simulink library "inp"  (R2021b)
settings: Solver=VariableStepAuto  StartTime=0.0  StopTime=10.0  RelTol=1e-3
undefined symbols (not defined in the file): C_TASK_5MS_S, FALSE, KINP_AcoreReadyToSlp_flg_ovrdflg, KINP_AcoreReadyToSlp_flg_ovrdval, KINP_AllowMovThd_OTA_enum_ovrdflg, KINP_AllowMovThd_OTA_enum_ovrdval, KINP_APSAngleTarget_Deg_ovrdflg, KINP_APSAngleTarget_Deg_ovrdval, KINP_APSDecReq_mps2_ovrdflg, KINP_APSDecReq_mps2_ovrdval, KINP_APSDecReqA_flg_ovrdflg, KINP_APSDecReqA_flg_ovrdval, KINP_APSDFLL_cm_ovrdflg, KINP_APSDFLL_cm_ovrdval, KINP_APSDFLR_cm_ovrdflg, KINP_APSDFLR_cm_ovrdval, KINP_APSDRLL_cm_ovrdflg, KINP_APSDRLL_cm_ovrdval, KINP_APSDRLR_cm_ovrdflg, KINP_APSDRLR_cm_ovrdval, KINP_APSExitCondition_enum_ovrdflg, KINP_APSExitCondition_enum_ovrdval, KINP_APSHWVer_enum_ovrdflg, KINP_APSHWVer_enum_ovrdval, KINP_APSProgressPCT_pct_ovrdflg, KINP_APSProgressPCT_pct_ovrdval, KINP_APSReq_enum_ovrdflg, KINP_APSReq_enum_ovrdval, KINP_APSRQDisplay_enum_ovrdflg, KINP_APSRQDisplay_enum_ovrdval, KINP_APSRqEPASCtrl_flg_ovrdflg, KINP_APSRqEPASCtrl_flg_ovrdval, KINP_APSShiftPosnReq_enum_ovrdval, KINP_APSShiftPosnReq_enum_ovrflg, KINP_APSSpeedCMD_kph_ovrdval, KINP_APSSpeedCMD_kph_ovrflg, KINP_APSStaSystem_enum_ovrdflg, KINP_APSStaSystem_enum_ovrdval, KINP_APSSWVer_enum_ovrdflg, KINP_APSSWVer_enum_ovrdval, KINP_APSVMCReqA_flg_ovrdval, KINP_APSVMCReqA_flg_ovrflg, KINP_APSVRqEPASCtrl_flg_ovrdflg, KINP_APSVRqEPASCtrl_flg_ovrdval, KINP_AuxBattVolmV_mV_ovrdflg, KINP_AuxBattVolmV_mV_ovrdval, KINP_CAASSta_enum_ovrdflg, KINP_CAASSta_enum_ovrdval, KINP_CAASVMCReqA_flg_ovrdval, KINP_CAASVMCReqA_flg_ovrflg, KINP_Chime_enum_ovrdflg, KINP_Chime_enum_ovrdval, KINP_ClearDTCcmd_flg_ovrdflg, KINP_ClearDTCcmd_flg_ovrdval, KINP_EvccAplusPwrUpReq_flg_ovrdflg, KINP_EvccAplusPwrUpReq_flg_ovrdval, KINP_LFID_raw_ovrdval, KINP_LFID_raw_ovrflg, KINP_LRID_raw_ovrdval, KINP_MemOffsetAccX_raw16_ovrdflg ... (+118)
libraries: FVT_lib x942, hcu_lib x1
(part 16 of 31)

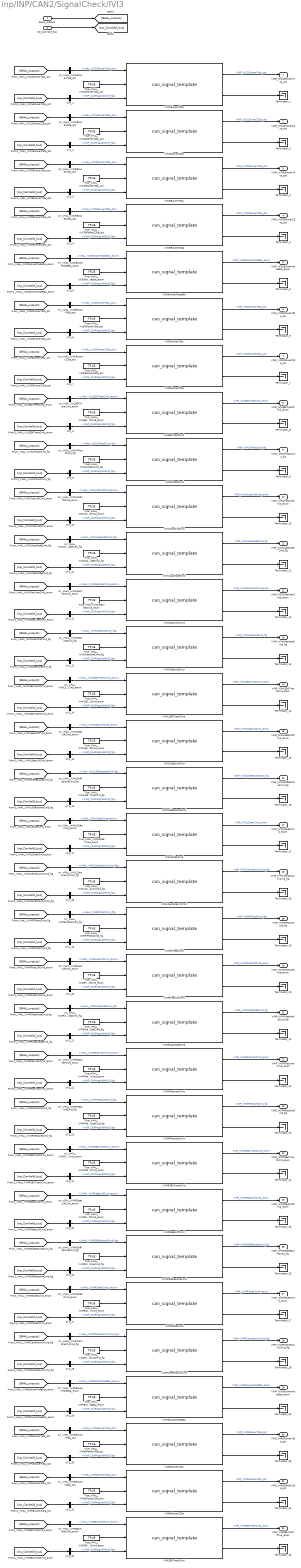
== system inp/INP/CAN2/SignalCheck/IVI3 ==
  BHAL_outputs : Inport
  inp_CanValid_bus : Inport  Port=2
  IVICLBlowerYSta : FVT_lib/inp/can_signal_template  SystemSampleTime=-1  VariantActivationTime=update diagram  Latency=0  AutoFrameSizeCalculation=off
      link override defval: Value=KINP_IVICLBlowerYSta_pct_defval
      link override ovrdflg: Value=KINP_IVICLBlowerYSta_pct_ovrdflg
      link override ovrdval: Value=KINP_IVICLBlowerYSta_pct_ovrdval
  IVICLBlowerZSta : FVT_lib/inp/can_signal_template  SystemSampleTime=-1  VariantActivationTime=update diagram  Latency=0  AutoFrameSizeCalculation=off
      link override defval: Value=KINP_IVICLBlowerZSta_pct_defval
      link override ovrdflg: Value=KINP_IVICLBlowerZSta_pct_ovrdflg
      link override ovrdval: Value=KINP_IVICLBlowerZSta_pct_ovrdval
  IVICRBlowerYSta : FVT_lib/inp/can_signal_template  SystemSampleTime=-1  VariantActivationTime=update diagram  Latency=0  AutoFrameSizeCalculation=off
      link override defval: Value=KINP_IVICRBlowerYSta_pct_defval
      link override ovrdflg: Value=KINP_IVICRBlowerYSta_pct_ovrdflg
      link override ovrdval: Value=KINP_IVICRBlowerYSta_pct_ovrdval
  IVICRBlowerZSta : FVT_lib/inp/can_signal_template  SystemSampleTime=-1  VariantActivationTime=update diagram  Latency=0  AutoFrameSizeCalculation=off
      link override defval: Value=KINP_IVICRBlowerZSta_pct_defval
      link override ovrdflg: Value=KINP_IVICRBlowerZSta_pct_ovrdflg
      link override ovrdval: Value=KINP_IVICRBlowerZSta_pct_ovrdval
  IVIDrBlowerModeSta : FVT_lib/inp/can_signal_template  SystemSampleTime=-1  VariantActivationTime=update diagram  Latency=0  AutoFrameSizeCalculation=off
      link override defval: Value=KINP_IVIDrBlowerModeSta_enum_defval
      link override ovrdflg: Value=KINP_IVIDrBlowerModeSta_enum_ovrdflg
      link override ovrdval: Value=KINP_IVIDrBlowerModeSta_enum_ovrdval
  IVIDrBlowerYSta : FVT_lib/inp/can_signal_template  SystemSampleTime=-1  VariantActivationTime=update diagram  Latency=0  AutoFrameSizeCalculation=off
      link override defval: Value=KINP_IVIDrBlowerYSta_pct_defval
      link override ovrdflg: Value=KINP_IVIDrBlowerYSta_pct_ovrdflg
      link override ovrdval: Value=KINP_IVIDrBlowerYSta_pct_ovrdval
  IVIDrBlowerZSta : FVT_lib/inp/can_signal_template  SystemSampleTime=-1  VariantActivationTime=update diagram  Latency=0  AutoFrameSizeCalculation=off
      link override defval: Value=KINP_IVIDrBlowerZSta_pct_defval
      link override ovrdflg: Value=KINP_IVIDrBlowerZSta_pct_ovrdflg
      link override ovrdval: Value=KINP_IVIDrBlowerZSta_pct_ovrdval
  IVILSEATventCmd : FVT_lib/inp/can_signal_template  SystemSampleTime=-1  VariantActivationTime=update diagram  Latency=0  AutoFrameSizeCalculation=off
      link override defval: Value=KINP_IVILSEATventCmd_enum_defval
      link override ovrdflg: Value=KINP_IVILSEATventCmd_enum_ovrdflg
      link override ovrdval: Value=KINP_IVILSEATventCmd_enum_ovrdval
  IVIMLFMostCmd : FVT_lib/inp/can_signal_template  SystemSampleTime=-1  VariantActivationTime=update diagram  Latency=0  AutoFrameSizeCalculation=off
      link override defval: Value=KINP_IVIMLFMostCmd_flg_defval
      link override ovrdflg: Value=KINP_IVIMLFMostCmd_flg_ovrdflg
      link override ovrdval: Value=KINP_IVIMLFMostCmd_flg_ovrdval
  IVIMLFootLiftCmd : FVT_lib/inp/can_signal_template  SystemSampleTime=-1  VariantActivationTime=update diagram  Latency=0  AutoFrameSizeCalculation=off
      link override defval: Value=KINP_IVIMLFootLiftCmd_enum_defval
      link override ovrdflg: Value=KINP_IVIMLFootLiftCmd_enum_ovrdflg
      link override ovrdval: Value=KINP_IVIMLFootLiftCmd_enum_ovrdval
  IVIMLNapModeCmd : FVT_lib/inp/can_signal_template  SystemSampleTime=-1  VariantActivationTime=update diagram  Latency=0  AutoFrameSizeCalculation=off
      link override defval: Value=KINP_IVIMLNapModeCmd_flg_defval
      link override ovrdflg: Value=KINP_IVIMLNapModeCmd_flg_ovrdflg
      link override ovrdval: Value=KINP_IVIMLNapModeCmd_flg_ovrdval
  IVIMLReclinerCmd : FVT_lib/inp/can_signal_template  SystemSampleTime=-1  VariantActivationTime=update diagram  Latency=0  AutoFrameSizeCalculation=off
      link override defval: Value=KINP_IVIMLReclinerCmd_enum_defval
      link override ovrdflg: Value=KINP_IVIMLReclinerCmd_enum_ovrdflg
      link override ovrdval: Value=KINP_IVIMLReclinerCmd_enum_ovrdval
  IVIMLRestoreCmd : FVT_lib/inp/can_signal_template  SystemSampleTime=-1  VariantActivationTime=update diagram  Latency=0  AutoFrameSizeCalculation=off
      link override defval: Value=KINP_IVIMLRestoreCmd_flg_defval
      link override ovrdflg: Value=KINP_IVIMLRestoreCmd_flg_ovrdflg
      link override ovrdval: Value=KINP_IVIMLRestoreCmd_flg_ovrdval
  IVIMLSEATventCmd : FVT_lib/inp/can_signal_template  SystemSampleTime=-1  VariantActivationTime=update diagram  Latency=0  AutoFrameSizeCalculation=off
      link override defval: Value=KINP_IVIMLSEATventCmd_enum_defval
      link override ovrdflg: Value=KINP_IVIMLSEATventCmd_enum_ovrdflg
      link override ovrdval: Value=KINP_IVIMLSEATventCmd_enum_ovrdval
  IVIMLSeatLiftCmd : FVT_lib/inp/can_signal_template  SystemSampleTime=-1  VariantActivationTime=update diagram  Latency=0  AutoFrameSizeCalculation=off
      link override defval: Value=KINP_IVIMLSeatLiftCmd_enum_defval
      link override ovrdflg: Value=KINP_IVIMLSeatLiftCmd_enum_ovrdflg
      link override ovrdval: Value=KINP_IVIMLSeatLiftCmd_enum_ovrdval
  IVIMLSldRestoreCmd : FVT_lib/inp/can_signal_template  SystemSampleTime=-1  VariantActivationTime=update diagram  Latency=0  AutoFrameSizeCalculation=off
      link override defval: Value=KINP_IVIMLSldRestoreCmd_flg_defval
      link override ovrdflg: Value=KINP_IVIMLSldRestoreCmd_flg_ovrdflg
      link override ovrdval: Value=KINP_IVIMLSldRestoreCmd_flg_ovrdval
  IVIMLSliderCmd : FVT_lib/inp/can_signal_template  SystemSampleTime=-1  VariantActivationTime=update diagram  Latency=0  AutoFrameSizeCalculation=off
      link override defval: Value=KINP_IVIMLSliderCmd_enum_defval
      link override ovrdflg: Value=KINP_IVIMLSliderCmd_enum_ovrdflg
      link override ovrdval: Value=KINP_IVIMLSliderCmd_enum_ovrdval
  IVIMLZeroGravityCmd : FVT_lib/inp/can_signal_template  SystemSampleTime=-1  VariantActivationTime=update diagram  Latency=0  AutoFrameSizeCalculation=off
      link override defval: Value=KINP_IVIMLZeroGravityCmd_flg_defval
      link override ovrdflg: Value=KINP_IVIMLZeroGravityCmd_flg_ovrdflg
      link override ovrdval: Value=KINP_IVIMLZeroGravityCmd_flg_ovrdval
  IVIMRFMostCmd : FVT_lib/inp/can_signal_template  SystemSampleTime=-1  VariantActivationTime=update diagram  Latency=0  AutoFrameSizeCalculation=off
      link override defval: Value=KINP_IVIMRFMostCmd_flg_defval
      link override ovrdflg: Value=KINP_IVIMRFMostCmd_flg_ovrdflg
      link override ovrdval: Value=KINP_IVIMRFMostCmd_flg_ovrdval
  IVIMRFootLiftCmd : FVT_lib/inp/can_signal_template  SystemSampleTime=-1  VariantActivationTime=update diagram  Latency=0  AutoFrameSizeCalculation=off
      link override defval: Value=KINP_IVIMRFootLiftCmd_enum_defval
      link override ovrdflg: Value=KINP_IVIMRFootLiftCmd_enum_ovrdflg
      link override ovrdval: Value=KINP_IVIMRFootLiftCmd_enum_ovrdval
  IVIMRNapModeCmd : FVT_lib/inp/can_signal_template  SystemSampleTime=-1  VariantActivationTime=update diagram  Latency=0  AutoFrameSizeCalculation=off
      link override defval: Value=KINP_IVIMRNapModeCmd_flg_defval
      link override ovrdflg: Value=KINP_IVIMRNapModeCmd_flg_ovrdflg
      link override ovrdval: Value=KINP_IVIMRNapModeCmd_flg_ovrdval
  IVIMRReclinerCmd : FVT_lib/inp/can_signal_template  SystemSampleTime=-1  VariantActivationTime=update diagram  Latency=0  AutoFrameSizeCalculation=off
      link override defval: Value=KINP_IVIMRReclinerCmd_enum_defval
      link override ovrdflg: Value=KINP_IVIMRReclinerCmd_enum_ovrdflg
      link override ovrdval: Value=KINP_IVIMRReclinerCmd_enum_ovrdval
  IVIMRRestoreCmd : FVT_lib/inp/can_signal_template  SystemSampleTime=-1  VariantActivationTime=update diagram  Latency=0  AutoFrameSizeCalculation=off
      link override defval: Value=KINP_IVIMRRestoreCmd_flg_defval
      link override ovrdflg: Value=KINP_IVIMRRestoreCmd_flg_ovrdflg
      link override ovrdval: Value=KINP_IVIMRRestoreCmd_flg_ovrdval
  IVIMRSEATventCmd : FVT_lib/inp/can_signal_template  SystemSampleTime=-1  VariantActivationTime=update diagram  Latency=0  AutoFrameSizeCalculation=off
      link override defval: Value=KINP_IVIMRSEATventCmd_enum_defval
      link override ovrdflg: Value=KINP_IVIMRSEATventCmd_enum_ovrdflg
      link override ovrdval: Value=KINP_IVIMRSEATventCmd_enum_ovrdval
  IVIMRSeatLiftCmd : FVT_lib/inp/can_signal_template  SystemSampleTime=-1  VariantActivationTime=update diagram  Latency=0  AutoFrameSizeCalculation=off
      link override defval: Value=KINP_IVIMRSeatLiftCmd_enum_defval
      link override ovrdflg: Value=KINP_IVIMRSeatLiftCmd_enum_ovrdflg
      link override ovrdval: Value=KINP_IVIMRSeatLiftCmd_enum_ovrdval
  IVIMRSldRestoreCmd : FVT_lib/inp/can_signal_template  SystemSampleTime=-1  VariantActivationTime=update diagram  Latency=0  AutoFrameSizeCalculation=off
      link override defval: Value=KINP_IVIMRSldRestoreCmd_flg_defval
      link override ovrdflg: Value=KINP_IVIMRSldRestoreCmd_flg_ovrdflg
      link override ovrdval: Value=KINP_IVIMRSldRestoreCmd_flg_ovrdval
  IVIMRSliderCmd : FVT_lib/inp/can_signal_template  SystemSampleTime=-1  VariantActivationTime=update diagram  Latency=0  AutoFrameSizeCalculation=off
      link override defval: Value=KINP_IVIMRSliderCmd_enum_defval
      link override ovrdflg: Value=KINP_IVIMRSliderCmd_enum_ovrdflg
      link override ovrdval: Value=KINP_IVIMRSliderCmd_enum_ovrdval
  IVIMRZeroGravityCmd : FVT_lib/inp/can_signal_template  SystemSampleTime=-1  VariantActivationTime=update diagram  Latency=0  AutoFrameSizeCalculation=off
      link override defval: Value=KINP_IVIMRZeroGravityCmd_flg_defval
      link override ovrdflg: Value=KINP_IVIMRZeroGravityCmd_flg_ovrdflg
      link override ovrdval: Value=KINP_IVIMRZeroGravityCmd_flg_ovrdval
  IVIPsBlowerModeSta : FVT_lib/inp/can_signal_template  SystemSampleTime=-1  VariantActivationTime=update diagram  Latency=0  AutoFrameSizeCalculation=off
      link override defval: Value=KINP_IVIPsBlowerModeSta_enum_defval
      link override ovrdflg: Value=KINP_IVIPsBlowerModeSta_enum_ovrdflg
      link override ovrdval: Value=KINP_IVIPsBlowerModeSta_enum_ovrdval
  IVIPsBlowerYSta : FVT_lib/inp/can_signal_template  SystemSampleTime=-1  VariantActivationTime=update diagram  Latency=0  AutoFrameSizeCalculation=off
      link override defval: Value=KINP_IVIPsBlowerYSta_pct_defval
      link override ovrdflg: Value=KINP_IVIPsBlowerYSta_pct_ovrdflg
      link override ovrdval: Value=KINP_IVIPsBlowerYSta_pct_ovrdval
  IVIPsBlowerZSta : FVT_lib/inp/can_signal_template  SystemSampleTime=-1  VariantActivationTime=update diagram  Latency=0  AutoFrameSizeCalculation=off
      link override defval: Value=KINP_IVIPsBlowerZSta_pct_defval
      link override ovrdflg: Value=KINP_IVIPsBlowerZSta_pct_ovrdflg
      link override ovrdval: Value=KINP_IVIPsBlowerZSta_pct_ovrdval
  IVIRSEATventCmd : FVT_lib/inp/can_signal_template  SystemSampleTime=-1  VariantActivationTime=update diagram  Latency=0  AutoFrameSizeCalculation=off
      link override defval: Value=KINP_IVIRSEATventCmd_enum_defval
      link override ovrdflg: Value=KINP_IVIRSEATventCmd_enum_ovrdflg
      link override ovrdval: Value=KINP_IVIRSEATventCmd_enum_ovrdval
  Terminator_{1..32} (32 alike) : Terminator
  True_VHAL_IVICLBlowerYSta_pct : Constant  Value=TRUE  OutDataTypeStr=boolean
  True_VHAL_IVICLBlowerZSta_pct : Constant  Value=TRUE  OutDataTypeStr=boolean
  True_VHAL_IVICRBlowerYSta_pct : Constant  Value=TRUE  OutDataTypeStr=boolean
  True_VHAL_IVICRBlowerZSta_pct : Constant  Value=TRUE  OutDataTypeStr=boolean
  True_VHAL_IVIDrBlowerModeSta_enum : Constant  Value=TRUE  OutDataTypeStr=boolean
  True_VHAL_IVIDrBlowerYSta_pct : Constant  Value=TRUE  OutDataTypeStr=boolean
  True_VHAL_IVIDrBlowerZSta_pct : Constant  Value=TRUE  OutDataTypeStr=boolean
  True_VHAL_IVILSEATventCmd_enum : Constant  Value=TRUE  OutDataTypeStr=boolean
  True_VHAL_IVIMLFMostCmd_flg : Constant  Value=TRUE  OutDataTypeStr=boolean
  True_VHAL_IVIMLFootLiftCmd_enum : Constant  Value=TRUE  OutDataTypeStr=boolean
  True_VHAL_IVIMLNapModeCmd_flg : Constant  Value=TRUE  OutDataTypeStr=boolean
  True_VHAL_IVIMLReclinerCmd_enum : Constant  Value=TRUE  OutDataTypeStr=boolean
  True_VHAL_IVIMLRestoreCmd_flg : Constant  Value=TRUE  OutDataTypeStr=boolean
  True_VHAL_IVIMLSEATventCmd_enum : Constant  Value=TRUE  OutDataTypeStr=boolean
  True_VHAL_IVIMLSeatLiftCmd_enum : Constant  Value=TRUE  OutDataTypeStr=boolean
  True_VHAL_IVIMLSldRestoreCmd_flg : Constant  Value=TRUE  OutDataTypeStr=boolean
  True_VHAL_IVIMLSliderCmd_enum : Constant  Value=TRUE  OutDataTypeStr=boolean
  True_VHAL_IVIMLZeroGravityCmd_flg : Constant  Value=TRUE  OutDataTypeStr=boolean
  True_VHAL_IVIMRFMostCmd_flg : Constant  Value=TRUE  OutDataTypeStr=boolean
  True_VHAL_IVIMRFootLiftCmd_enum : Constant  Value=TRUE  OutDataTypeStr=boolean
  True_VHAL_IVIMRNapModeCmd_flg : Constant  Value=TRUE  OutDataTypeStr=boolean
  True_VHAL_IVIMRReclinerCmd_enum : Constant  Value=TRUE  OutDataTypeStr=boolean
  True_VHAL_IVIMRRestoreCmd_flg : Constant  Value=TRUE  OutDataTypeStr=boolean
  True_VHAL_IVIMRSEATventCmd_enum : Constant  Value=TRUE  OutDataTypeStr=boolean
  True_VHAL_IVIMRSeatLiftCmd_enum : Constant  Value=TRUE  OutDataTypeStr=boolean
  True_VHAL_IVIMRSldRestoreCmd_flg : Constant  Value=TRUE  OutDataTypeStr=boolean
  True_VHAL_IVIMRSliderCmd_enum : Constant  Value=TRUE  OutDataTypeStr=boolean
  True_VHAL_IVIMRZeroGravityCmd_flg : Constant  Value=TRUE  OutDataTypeStr=boolean
  True_VHAL_IVIPsBlowerModeSta_enum : Constant  Value=TRUE  OutDataTypeStr=boolean
  True_VHAL_IVIPsBlowerYSta_pct : Constant  Value=TRUE  OutDataTypeStr=boolean
  True_VHAL_IVIPsBlowerZSta_pct : Constant  Value=TRUE  OutDataTypeStr=boolean
  True_VHAL_IVIRSEATventCmd_enum : Constant  Value=TRUE  OutDataTypeStr=boolean
  slr1_{1..32} (32 alike) : BusSelector  OutputSignals=VINP_CANMsgValidIVI3_flg
  slr_VHAL_IVICLBlowerYSta_pct : BusSelector  OutputSignals=VHAL_IVICLBlowerYSta_pct
  slr_VHAL_IVICLBlowerZSta_pct : BusSelector  OutputSignals=VHAL_IVICLBlowerZSta_pct
  slr_VHAL_IVICRBlowerYSta_pct : BusSelector  OutputSignals=VHAL_IVICRBlowerYSta_pct
  slr_VHAL_IVICRBlowerZSta_pct : BusSelector  OutputSignals=VHAL_IVICRBlowerZSta_pct
  slr_VHAL_IVIDrBlowerModeSta_enum : BusSelector  OutputSignals=VHAL_IVIDrBlowerModeSta_enum
  slr_VHAL_IVIDrBlowerYSta_pct : BusSelector  OutputSignals=VHAL_IVIDrBlowerYSta_pct
  slr_VHAL_IVIDrBlowerZSta_pct : BusSelector  OutputSignals=VHAL_IVIDrBlowerZSta_pct
  slr_VHAL_IVILSEATventCmd_enum : BusSelector  OutputSignals=VHAL_IVILSEATventCmd_enum
  slr_VHAL_IVIMLFMostCmd_flg : BusSelector  OutputSignals=VHAL_IVIMLFMostCmd_flg
  slr_VHAL_IVIMLFootLiftCmd_enum : BusSelector  OutputSignals=VHAL_IVIMLFootLiftCmd_enum
  slr_VHAL_IVIMLNapModeCmd_flg : BusSelector  OutputSignals=VHAL_IVIMLNapModeCmd_flg
  slr_VHAL_IVIMLReclinerCmd_enum : BusSelector  OutputSignals=VHAL_IVIMLReclinerCmd_enum
  slr_VHAL_IVIMLRestoreCmd_flg : BusSelector  OutputSignals=VHAL_IVIMLRestoreCmd_flg
  slr_VHAL_IVIMLSEATventCmd_enum : BusSelector  OutputSignals=VHAL_IVIMLSEATventCmd_enum
  slr_VHAL_IVIMLSeatLiftCmd_enum : BusSelector  OutputSignals=VHAL_IVIMLSeatLiftCmd_enum
  slr_VHAL_IVIMLSldRestoreCmd_flg : BusSelector  OutputSignals=VHAL_IVIMLSldRestoreCmd_flg
  slr_VHAL_IVIMLSliderCmd_enum : BusSelector  OutputSignals=VHAL_IVIMLSliderCmd_enum
  slr_VHAL_IVIMLZeroGravityCmd_flg : BusSelector  OutputSignals=VHAL_IVIMLZeroGravityCmd_flg
  slr_VHAL_IVIMRFMostCmd_flg : BusSelector  OutputSignals=VHAL_IVIMRFMostCmd_flg
  slr_VHAL_IVIMRFootLiftCmd_enum : BusSelector  OutputSignals=VHAL_IVIMRFootLiftCmd_enum
  slr_VHAL_IVIMRNapModeCmd_flg : BusSelector  OutputSignals=VHAL_IVIMRNapModeCmd_flg
  slr_VHAL_IVIMRReclinerCmd_enum : BusSelector  OutputSignals=VHAL_IVIMRReclinerCmd_enum
  slr_VHAL_IVIMRRestoreCmd_flg : BusSelector  OutputSignals=VHAL_IVIMRRestoreCmd_flg
  slr_VHAL_IVIMRSEATventCmd_enum : BusSelector  OutputSignals=VHAL_IVIMRSEATventCmd_enum
  slr_VHAL_IVIMRSeatLiftCmd_enum : BusSelector  OutputSignals=VHAL_IVIMRSeatLiftCmd_enum
  slr_VHAL_IVIMRSldRestoreCmd_flg : BusSelector  OutputSignals=VHAL_IVIMRSldRestoreCmd_flg
  slr_VHAL_IVIMRSliderCmd_enum : BusSelector  OutputSignals=VHAL_IVIMRSliderCmd_enum
  slr_VHAL_IVIMRZeroGravityCmd_flg : BusSelector  OutputSignals=VHAL_IVIMRZeroGravityCmd_flg
  slr_VHAL_IVIPsBlowerModeSta_enum : BusSelector  OutputSignals=VHAL_IVIPsBlowerModeSta_enum
  slr_VHAL_IVIPsBlowerYSta_pct : BusSelector  OutputSignals=VHAL_IVIPsBlowerYSta_pct
  slr_VHAL_IVIPsBlowerZSta_pct : BusSelector  OutputSignals=VHAL_IVIPsBlowerZSta_pct
  slr_VHAL_IVIRSEATventCmd_enum : BusSelector  OutputSignals=VHAL_IVIRSEATventCmd_enum
  VINP_IVICLBlowerYSta_pct : Outport
  VINP_IVICLBlowerZSta_pct : Outport  Port=2
  VINP_IVICRBlowerYSta_pct : Outport  Port=3
  VINP_IVICRBlowerZSta_pct : Outport  Port=4
  VINP_IVIDrBlowerModeSta_enum : Outport  Port=5
  VINP_IVIDrBlowerYSta_pct : Outport  Port=6
  VINP_IVIDrBlowerZSta_pct : Outport  Port=7
  VINP_IVILSEATventCmd_enum : Outport  Port=8
  VINP_IVIMLFMostCmd_flg : Outport  Port=9
  VINP_IVIMLFootLiftCmd_enum : Outport  Port=10
  VINP_IVIMLNapModeCmd_flg : Outport  Port=11
  VINP_IVIMLReclinerCmd_enum : Outport  Port=12
  VINP_IVIMLRestoreCmd_flg : Outport  Port=13
  VINP_IVIMLSEATventCmd_enum : Outport  Port=14
  VINP_IVIMLSeatLiftCmd_enum : Outport  Port=15
  VINP_IVIMLSldRestoreCmd_flg : Outport  Port=16
  VINP_IVIMLSliderCmd_enum : Outport  Port=17
  VINP_IVIMLZeroGravityCmd_flg : Outport  Port=18
  VINP_IVIMRFMostCmd_flg : Outport  Port=19
  VINP_IVIMRFootLiftCmd_enum : Outport  Port=20
  VINP_IVIMRNapModeCmd_flg : Outport  Port=21
  VINP_IVIMRReclinerCmd_enum : Outport  Port=22
  VINP_IVIMRRestoreCmd_flg : Outport  Port=23
  VINP_IVIMRSEATventCmd_enum : Outport  Port=24
  VINP_IVIMRSeatLiftCmd_enum : Outport  Port=25
  VINP_IVIMRSldRestoreCmd_flg : Outport  Port=26
  VINP_IVIMRSliderCmd_enum : Outport  Port=27
  VINP_IVIMRZeroGravityCmd_flg : Outport  Port=28
  VINP_IVIPsBlowerModeSta_enum : Outport  Port=29
  VINP_IVIPsBlowerYSta_pct : Outport  Port=30
  VINP_IVIPsBlowerZSta_pct : Outport  Port=31
  VINP_IVIRSEATventCmd_enum : Outport  Port=32
  wires:
  BHAL_outputs/1 -> [BHAL_outputs]
  inp_CanValid_bus/1 -> [inp_CanValid_bus]
  [BHAL_outputs] -> slr_VHAL_IVICLBlowerYSta_pct/1
  slr_VHAL_IVICLBlowerYSta_pct/1 -> IVICLBlowerYSta/1  "<VHAL_IVICLBlowerYSta_pct>"
  True_VHAL_IVICLBlowerYSta_pct/1 -> IVICLBlowerYSta/2
  [inp_CanValid_bus] -> slr1_1/1
  slr1_1/1 -> IVICLBlowerYSta/3  "<VINP_CANMsgValidIVI3_flg>"
  IVICLBlowerYSta/1 -> VINP_IVICLBlowerYSta_pct/1  "VINP_IVICLBlowerYSta_pct"
  IVICLBlowerYSta/2 -> Terminator_1/1
  [BHAL_outputs] -> slr_VHAL_IVICLBlowerZSta_pct/1
  slr_VHAL_IVICLBlowerZSta_pct/1 -> IVICLBlowerZSta/1  "<VHAL_IVICLBlowerZSta_pct>"
  True_VHAL_IVICLBlowerZSta_pct/1 -> IVICLBlowerZSta/2
  [inp_CanValid_bus] -> slr1_2/1
  slr1_2/1 -> IVICLBlowerZSta/3  "<VINP_CANMsgValidIVI3_flg>"
  IVICLBlowerZSta/1 -> VINP_IVICLBlowerZSta_pct/1  "VINP_IVICLBlowerZSta_pct"
  IVICLBlowerZSta/2 -> Terminator_2/1
  [BHAL_outputs] -> slr_VHAL_IVICRBlowerYSta_pct/1
  slr_VHAL_IVICRBlowerYSta_pct/1 -> IVICRBlowerYSta/1  "<VHAL_IVICRBlowerYSta_pct>"
  True_VHAL_IVICRBlowerYSta_pct/1 -> IVICRBlowerYSta/2
  [inp_CanValid_bus] -> slr1_3/1
  slr1_3/1 -> IVICRBlowerYSta/3  "<VINP_CANMsgValidIVI3_flg>"
  IVICRBlowerYSta/1 -> VINP_IVICRBlowerYSta_pct/1  "VINP_IVICRBlowerYSta_pct"
  IVICRBlowerYSta/2 -> Terminator_3/1
  [BHAL_outputs] -> slr_VHAL_IVICRBlowerZSta_pct/1
  slr_VHAL_IVICRBlowerZSta_pct/1 -> IVICRBlowerZSta/1  "<VHAL_IVICRBlowerZSta_pct>"
  True_VHAL_IVICRBlowerZSta_pct/1 -> IVICRBlowerZSta/2
  [inp_CanValid_bus] -> slr1_4/1
  slr1_4/1 -> IVICRBlowerZSta/3  "<VINP_CANMsgValidIVI3_flg>"
  IVICRBlowerZSta/1 -> VINP_IVICRBlowerZSta_pct/1  "VINP_IVICRBlowerZSta_pct"
  IVICRBlowerZSta/2 -> Terminator_4/1
  [BHAL_outputs] -> slr_VHAL_IVIDrBlowerModeSta_enum/1
  slr_VHAL_IVIDrBlowerModeSta_enum/1 -> IVIDrBlowerModeSta/1  "<VHAL_IVIDrBlowerModeSta_enum>"
  True_VHAL_IVIDrBlowerModeSta_enum/1 -> IVIDrBlowerModeSta/2
  [inp_CanValid_bus] -> slr1_5/1
  slr1_5/1 -> IVIDrBlowerModeSta/3  "<VINP_CANMsgValidIVI3_flg>"
  IVIDrBlowerModeSta/1 -> VINP_IVIDrBlowerModeSta_enum/1  "VINP_IVIDrBlowerModeSta_enum"
  IVIDrBlowerModeSta/2 -> Terminator_5/1
  [BHAL_outputs] -> slr_VHAL_IVIDrBlowerYSta_pct/1
  slr_VHAL_IVIDrBlowerYSta_pct/1 -> IVIDrBlowerYSta/1  "<VHAL_IVIDrBlowerYSta_pct>"
  True_VHAL_IVIDrBlowerYSta_pct/1 -> IVIDrBlowerYSta/2
  [inp_CanValid_bus] -> slr1_6/1
  slr1_6/1 -> IVIDrBlowerYSta/3  "<VINP_CANMsgValidIVI3_flg>"
  IVIDrBlowerYSta/1 -> VINP_IVIDrBlowerYSta_pct/1  "VINP_IVIDrBlowerYSta_pct"
  IVIDrBlowerYSta/2 -> Terminator_6/1
  [BHAL_outputs] -> slr_VHAL_IVIDrBlowerZSta_pct/1
  slr_VHAL_IVIDrBlowerZSta_pct/1 -> IVIDrBlowerZSta/1  "<VHAL_IVIDrBlowerZSta_pct>"
  True_VHAL_IVIDrBlowerZSta_pct/1 -> IVIDrBlowerZSta/2
  [inp_CanValid_bus] -> slr1_7/1
  slr1_7/1 -> IVIDrBlowerZSta/3  "<VINP_CANMsgValidIVI3_flg>"
  IVIDrBlowerZSta/1 -> VINP_IVIDrBlowerZSta_pct/1  "VINP_IVIDrBlowerZSta_pct"
  IVIDrBlowerZSta/2 -> Terminator_7/1
  [BHAL_outputs] -> slr_VHAL_IVILSEATventCmd_enum/1
  slr_VHAL_IVILSEATventCmd_enum/1 -> IVILSEATventCmd/1  "<VHAL_IVILSEATventCmd_enum>"
  True_VHAL_IVILSEATventCmd_enum/1 -> IVILSEATventCmd/2
  [inp_CanValid_bus] -> slr1_8/1
  slr1_8/1 -> IVILSEATventCmd/3  "<VINP_CANMsgValidIVI3_flg>"
  IVILSEATventCmd/1 -> VINP_IVILSEATventCmd_enum/1  "VINP_IVILSEATventCmd_enum"
  IVILSEATventCmd/2 -> Terminator_8/1
  [BHAL_outputs] -> slr_VHAL_IVIMLFMostCmd_flg/1
  slr_VHAL_IVIMLFMostCmd_flg/1 -> IVIMLFMostCmd/1  "<VHAL_IVIMLFMostCmd_flg>"
  True_VHAL_IVIMLFMostCmd_flg/1 -> IVIMLFMostCmd/2
  [inp_CanValid_bus] -> slr1_9/1
  slr1_9/1 -> IVIMLFMostCmd/3  "<VINP_CANMsgValidIVI3_flg>"
  IVIMLFMostCmd/1 -> VINP_IVIMLFMostCmd_flg/1  "VINP_IVIMLFMostCmd_flg"
  IVIMLFMostCmd/2 -> Terminator_9/1
  [BHAL_outputs] -> slr_VHAL_IVIMLFootLiftCmd_enum/1
  slr_VHAL_IVIMLFootLiftCmd_enum/1 -> IVIMLFootLiftCmd/1  "<VHAL_IVIMLFootLiftCmd_enum>"
  True_VHAL_IVIMLFootLiftCmd_enum/1 -> IVIMLFootLiftCmd/2
  [inp_CanValid_bus] -> slr1_10/1
  slr1_10/1 -> IVIMLFootLiftCmd/3  "<VINP_CANMsgValidIVI3_flg>"
  IVIMLFootLiftCmd/1 -> VINP_IVIMLFootLiftCmd_enum/1  "VINP_IVIMLFootLiftCmd_enum"
  IVIMLFootLiftCmd/2 -> Terminator_10/1
  [BHAL_outputs] -> slr_VHAL_IVIMLNapModeCmd_flg/1
  slr_VHAL_IVIMLNapModeCmd_flg/1 -> IVIMLNapModeCmd/1  "<VHAL_IVIMLNapModeCmd_flg>"
  True_VHAL_IVIMLNapModeCmd_flg/1 -> IVIMLNapModeCmd/2
  [inp_CanValid_bus] -> slr1_11/1
  slr1_11/1 -> IVIMLNapModeCmd/3  "<VINP_CANMsgValidIVI3_flg>"
  IVIMLNapModeCmd/1 -> VINP_IVIMLNapModeCmd_flg/1  "VINP_IVIMLNapModeCmd_flg"
  IVIMLNapModeCmd/2 -> Terminator_11/1
  [BHAL_outputs] -> slr_VHAL_IVIMLReclinerCmd_enum/1
  slr_VHAL_IVIMLReclinerCmd_enum/1 -> IVIMLReclinerCmd/1  "<VHAL_IVIMLReclinerCmd_enum>"
  True_VHAL_IVIMLReclinerCmd_enum/1 -> IVIMLReclinerCmd/2
  [inp_CanValid_bus] -> slr1_12/1
  slr1_12/1 -> IVIMLReclinerCmd/3  "<VINP_CANMsgValidIVI3_flg>"
  IVIMLReclinerCmd/1 -> VINP_IVIMLReclinerCmd_enum/1  "VINP_IVIMLReclinerCmd_enum"
  IVIMLReclinerCmd/2 -> Terminator_12/1
  [BHAL_outputs] -> slr_VHAL_IVIMLRestoreCmd_flg/1
  slr_VHAL_IVIMLRestoreCmd_flg/1 -> IVIMLRestoreCmd/1  "<VHAL_IVIMLRestoreCmd_flg>"
  True_VHAL_IVIMLRestoreCmd_flg/1 -> IVIMLRestoreCmd/2
  [inp_CanValid_bus] -> slr1_13/1
  slr1_13/1 -> IVIMLRestoreCmd/3  "<VINP_CANMsgValidIVI3_flg>"
  IVIMLRestoreCmd/1 -> VINP_IVIMLRestoreCmd_flg/1  "VINP_IVIMLRestoreCmd_flg"
  IVIMLRestoreCmd/2 -> Terminator_13/1
  [BHAL_outputs] -> slr_VHAL_IVIMLSEATventCmd_enum/1
  slr_VHAL_IVIMLSEATventCmd_enum/1 -> IVIMLSEATventCmd/1  "<VHAL_IVIMLSEATventCmd_enum>"
  True_VHAL_IVIMLSEATventCmd_enum/1 -> IVIMLSEATventCmd/2
  [inp_CanValid_bus] -> slr1_14/1
  slr1_14/1 -> IVIMLSEATventCmd/3  "<VINP_CANMsgValidIVI3_flg>"
  IVIMLSEATventCmd/1 -> VINP_IVIMLSEATventCmd_enum/1  "VINP_IVIMLSEATventCmd_enum"
  IVIMLSEATventCmd/2 -> Terminator_14/1
  [BHAL_outputs] -> slr_VHAL_IVIMLSeatLiftCmd_enum/1
  slr_VHAL_IVIMLSeatLiftCmd_enum/1 -> IVIMLSeatLiftCmd/1  "<VHAL_IVIMLSeatLiftCmd_enum>"
  True_VHAL_IVIMLSeatLiftCmd_enum/1 -> IVIMLSeatLiftCmd/2
  [inp_CanValid_bus] -> slr1_15/1
  slr1_15/1 -> IVIMLSeatLiftCmd/3  "<VINP_CANMsgValidIVI3_flg>"
  IVIMLSeatLiftCmd/1 -> VINP_IVIMLSeatLiftCmd_enum/1  "VINP_IVIMLSeatLiftCmd_enum"
  IVIMLSeatLiftCmd/2 -> Terminator_15/1
  [BHAL_outputs] -> slr_VHAL_IVIMLSldRestoreCmd_flg/1
  slr_VHAL_IVIMLSldRestoreCmd_flg/1 -> IVIMLSldRestoreCmd/1  "<VHAL_IVIMLSldRestoreCmd_flg>"
  True_VHAL_IVIMLSldRestoreCmd_flg/1 -> IVIMLSldRestoreCmd/2
  [inp_CanValid_bus] -> slr1_16/1
  slr1_16/1 -> IVIMLSldRestoreCmd/3  "<VINP_CANMsgValidIVI3_flg>"
  IVIMLSldRestoreCmd/1 -> VINP_IVIMLSldRestoreCmd_flg/1  "VINP_IVIMLSldRestoreCmd_flg"
  IVIMLSldRestoreCmd/2 -> Terminator_16/1
  [BHAL_outputs] -> slr_VHAL_IVIMLSliderCmd_enum/1
  slr_VHAL_IVIMLSliderCmd_enum/1 -> IVIMLSliderCmd/1  "<VHAL_IVIMLSliderCmd_enum>"
  True_VHAL_IVIMLSliderCmd_enum/1 -> IVIMLSliderCmd/2
  [inp_CanValid_bus] -> slr1_17/1
  slr1_17/1 -> IVIMLSliderCmd/3  "<VINP_CANMsgValidIVI3_flg>"
  IVIMLSliderCmd/1 -> VINP_IVIMLSliderCmd_enum/1  "VINP_IVIMLSliderCmd_enum"
  IVIMLSliderCmd/2 -> Terminator_17/1
  [BHAL_outputs] -> slr_VHAL_IVIMLZeroGravityCmd_flg/1
  slr_VHAL_IVIMLZeroGravityCmd_flg/1 -> IVIMLZeroGravityCmd/1  "<VHAL_IVIMLZeroGravityCmd_flg>"
  True_VHAL_IVIMLZeroGravityCmd_flg/1 -> IVIMLZeroGravityCmd/2
  [inp_CanValid_bus] -> slr1_18/1
  slr1_18/1 -> IVIMLZeroGravityCmd/3  "<VINP_CANMsgValidIVI3_flg>"
  IVIMLZeroGravityCmd/1 -> VINP_IVIMLZeroGravityCmd_flg/1  "VINP_IVIMLZeroGravityCmd_flg"
  IVIMLZeroGravityCmd/2 -> Terminator_18/1
  [BHAL_outputs] -> slr_VHAL_IVIMRFMostCmd_flg/1
  slr_VHAL_IVIMRFMostCmd_flg/1 -> IVIMRFMostCmd/1  "<VHAL_IVIMRFMostCmd_flg>"
  True_VHAL_IVIMRFMostCmd_flg/1 -> IVIMRFMostCmd/2
  [inp_CanValid_bus] -> slr1_19/1
  slr1_19/1 -> IVIMRFMostCmd/3  "<VINP_CANMsgValidIVI3_flg>"
  IVIMRFMostCmd/1 -> VINP_IVIMRFMostCmd_flg/1  "VINP_IVIMRFMostCmd_flg"
  IVIMRFMostCmd/2 -> Terminator_19/1
  [BHAL_outputs] -> slr_VHAL_IVIMRFootLiftCmd_enum/1
  slr_VHAL_IVIMRFootLiftCmd_enum/1 -> IVIMRFootLiftCmd/1  "<VHAL_IVIMRFootLiftCmd_enum>"
  True_VHAL_IVIMRFootLiftCmd_enum/1 -> IVIMRFootLiftCmd/2
  [inp_CanValid_bus] -> slr1_20/1
  slr1_20/1 -> IVIMRFootLiftCmd/3  "<VINP_CANMsgValidIVI3_flg>"
  IVIMRFootLiftCmd/1 -> VINP_IVIMRFootLiftCmd_enum/1  "VINP_IVIMRFootLiftCmd_enum"
  IVIMRFootLiftCmd/2 -> Terminator_20/1
  [BHAL_outputs] -> slr_VHAL_IVIMRNapModeCmd_flg/1
  slr_VHAL_IVIMRNapModeCmd_flg/1 -> IVIMRNapModeCmd/1  "<VHAL_IVIMRNapModeCmd_flg>"
  True_VHAL_IVIMRNapModeCmd_flg/1 -> IVIMRNapModeCmd/2
  [inp_CanValid_bus] -> slr1_21/1
  slr1_21/1 -> IVIMRNapModeCmd/3  "<VINP_CANMsgValidIVI3_flg>"
  IVIMRNapModeCmd/1 -> VINP_IVIMRNapModeCmd_flg/1  "VINP_IVIMRNapModeCmd_flg"
  IVIMRNapModeCmd/2 -> Terminator_21/1
  [BHAL_outputs] -> slr_VHAL_IVIMRReclinerCmd_enum/1
  slr_VHAL_IVIMRReclinerCmd_enum/1 -> IVIMRReclinerCmd/1  "<VHAL_IVIMRReclinerCmd_enum>"
  True_VHAL_IVIMRReclinerCmd_enum/1 -> IVIMRReclinerCmd/2
  [inp_CanValid_bus] -> slr1_22/1
  slr1_22/1 -> IVIMRReclinerCmd/3  "<VINP_CANMsgValidIVI3_flg>"
  IVIMRReclinerCmd/1 -> VINP_IVIMRReclinerCmd_enum/1  "VINP_IVIMRReclinerCmd_enum"
  IVIMRReclinerCmd/2 -> Terminator_22/1
  [BHAL_outputs] -> slr_VHAL_IVIMRRestoreCmd_flg/1
  slr_VHAL_IVIMRRestoreCmd_flg/1 -> IVIMRRestoreCmd/1  "<VHAL_IVIMRRestoreCmd_flg>"
  True_VHAL_IVIMRRestoreCmd_flg/1 -> IVIMRRestoreCmd/2
  [inp_CanValid_bus] -> slr1_23/1
  slr1_23/1 -> IVIMRRestoreCmd/3  "<VINP_CANMsgValidIVI3_flg>"
  IVIMRRestoreCmd/1 -> VINP_IVIMRRestoreCmd_flg/1  "VINP_IVIMRRestoreCmd_flg"
  IVIMRRestoreCmd/2 -> Terminator_23/1
  [BHAL_outputs] -> slr_VHAL_IVIMRSEATventCmd_enum/1
  slr_VHAL_IVIMRSEATventCmd_enum/1 -> IVIMRSEATventCmd/1  "<VHAL_IVIMRSEATventCmd_enum>"
  True_VHAL_IVIMRSEATventCmd_enum/1 -> IVIMRSEATventCmd/2
  [inp_CanValid_bus] -> slr1_24/1
  slr1_24/1 -> IVIMRSEATventCmd/3  "<VINP_CANMsgValidIVI3_flg>"
  IVIMRSEATventCmd/1 -> VINP_IVIMRSEATventCmd_enum/1  "VINP_IVIMRSEATventCmd_enum"
  IVIMRSEATventCmd/2 -> Terminator_24/1
  [BHAL_outputs] -> slr_VHAL_IVIMRSeatLiftCmd_enum/1
  slr_VHAL_IVIMRSeatLiftCmd_enum/1 -> IVIMRSeatLiftCmd/1  "<VHAL_IVIMRSeatLiftCmd_enum>"
  True_VHAL_IVIMRSeatLiftCmd_enum/1 -> IVIMRSeatLiftCmd/2
  [inp_CanValid_bus] -> slr1_25/1
  slr1_25/1 -> IVIMRSeatLiftCmd/3  "<VINP_CANMsgValidIVI3_flg>"
  IVIMRSeatLiftCmd/1 -> VINP_IVIMRSeatLiftCmd_enum/1  "VINP_IVIMRSeatLiftCmd_enum"
  IVIMRSeatLiftCmd/2 -> Terminator_25/1
  [BHAL_outputs] -> slr_VHAL_IVIMRSldRestoreCmd_flg/1
  slr_VHAL_IVIMRSldRestoreCmd_flg/1 -> IVIMRSldRestoreCmd/1  "<VHAL_IVIMRSldRestoreCmd_flg>"
  True_VHAL_IVIMRSldRestoreCmd_flg/1 -> IVIMRSldRestoreCmd/2
  [inp_CanValid_bus] -> slr1_26/1
  slr1_26/1 -> IVIMRSldRestoreCmd/3  "<VINP_CANMsgValidIVI3_flg>"
  IVIMRSldRestoreCmd/1 -> VINP_IVIMRSldRestoreCmd_flg/1  "VINP_IVIMRSldRestoreCmd_flg"
  IVIMRSldRestoreCmd/2 -> Terminator_26/1
  [BHAL_outputs] -> slr_VHAL_IVIMRSliderCmd_enum/1
  slr_VHAL_IVIMRSliderCmd_enum/1 -> IVIMRSliderCmd/1  "<VHAL_IVIMRSliderCmd_enum>"
  True_VHAL_IVIMRSliderCmd_enum/1 -> IVIMRSliderCmd/2
  [inp_CanValid_bus] -> slr1_27/1
  slr1_27/1 -> IVIMRSliderCmd/3  "<VINP_CANMsgValidIVI3_flg>"
  IVIMRSliderCmd/1 -> VINP_IVIMRSliderCmd_enum/1  "VINP_IVIMRSliderCmd_enum"
  IVIMRSliderCmd/2 -> Terminator_27/1
  [BHAL_outputs] -> slr_VHAL_IVIMRZeroGravityCmd_flg/1
  slr_VHAL_IVIMRZeroGravityCmd_flg/1 -> IVIMRZeroGravityCmd/1  "<VHAL_IVIMRZeroGravityCmd_flg>"
  True_VHAL_IVIMRZeroGravityCmd_flg/1 -> IVIMRZeroGravityCmd/2
  [inp_CanValid_bus] -> slr1_28/1
  slr1_28/1 -> IVIMRZeroGravityCmd/3  "<VINP_CANMsgValidIVI3_flg>"
  IVIMRZeroGravityCmd/1 -> VINP_IVIMRZeroGravityCmd_flg/1  "VINP_IVIMRZeroGravityCmd_flg"
  IVIMRZeroGravityCmd/2 -> Terminator_28/1
  [BHAL_outputs] -> slr_VHAL_IVIPsBlowerModeSta_enum/1
  slr_VHAL_IVIPsBlowerModeSta_enum/1 -> IVIPsBlowerModeSta/1  "<VHAL_IVIPsBlowerModeSta_enum>"
  True_VHAL_IVIPsBlowerModeSta_enum/1 -> IVIPsBlowerModeSta/2
  [inp_CanValid_bus] -> slr1_29/1
  slr1_29/1 -> IVIPsBlowerModeSta/3  "<VINP_CANMsgValidIVI3_flg>"
  IVIPsBlowerModeSta/1 -> VINP_IVIPsBlowerModeSta_enum/1  "VINP_IVIPsBlowerModeSta_enum"
  IVIPsBlowerModeSta/2 -> Terminator_29/1
  [BHAL_outputs] -> slr_VHAL_IVIPsBlowerYSta_pct/1
  slr_VHAL_IVIPsBlowerYSta_pct/1 -> IVIPsBlowerYSta/1  "<VHAL_IVIPsBlowerYSta_pct>"
  True_VHAL_IVIPsBlowerYSta_pct/1 -> IVIPsBlowerYSta/2
  [inp_CanValid_bus] -> slr1_30/1
  slr1_30/1 -> IVIPsBlowerYSta/3  "<VINP_CANMsgValidIVI3_flg>"
  IVIPsBlowerYSta/1 -> VINP_IVIPsBlowerYSta_pct/1  "VINP_IVIPsBlowerYSta_pct"
  IVIPsBlowerYSta/2 -> Terminator_30/1
  [BHAL_outputs] -> slr_VHAL_IVIPsBlowerZSta_pct/1
  slr_VHAL_IVIPsBlowerZSta_pct/1 -> IVIPsBlowerZSta/1  "<VHAL_IVIPsBlowerZSta_pct>"
  True_VHAL_IVIPsBlowerZSta_pct/1 -> IVIPsBlowerZSta/2
  [inp_CanValid_bus] -> slr1_31/1
  slr1_31/1 -> IVIPsBlowerZSta/3  "<VINP_CANMsgValidIVI3_flg>"
  IVIPsBlowerZSta/1 -> VINP_IVIPsBlowerZSta_pct/1  "VINP_IVIPsBlowerZSta_pct"
  IVIPsBlowerZSta/2 -> Terminator_31/1
  [BHAL_outputs] -> slr_VHAL_IVIRSEATventCmd_enum/1
  slr_VHAL_IVIRSEATventCmd_enum/1 -> IVIRSEATventCmd/1  "<VHAL_IVIRSEATventCmd_enum>"
  True_VHAL_IVIRSEATventCmd_enum/1 -> IVIRSEATventCmd/2
  [inp_CanValid_bus] -> slr1_32/1
  slr1_32/1 -> IVIRSEATventCmd/3  "<VINP_CANMsgValidIVI3_flg>"
  IVIRSEATventCmd/1 -> VINP_IVIRSEATventCmd_enum/1  "VINP_IVIRSEATventCmd_enum"
  IVIRSEATventCmd/2 -> Terminator_32/1

== system inp/INP/CAN2/SignalCheck/METER1 ==
  BHAL_outputs : Inport
  inp_CanValid_bus : Inport  Port=2
  METERKPHCalcu : FVT_lib/inp/can_signal_template  SystemSampleTime=-1  VariantActivationTime=update diagram  Latency=0  AutoFrameSizeCalculation=off
      link override defval: Value=KINP_METERKPHCalcu_kph_defval
      link override ovrdflg: Value=KINP_METERKPHCalcu_kph_ovrdflg
      link override ovrdval: Value=KINP_METERKPHCalcu_kph_ovrdval
  ODOMETER : FVT_lib/inp/can_signal_template  SystemSampleTime=-1  VariantActivationTime=update diagram  Latency=0  AutoFrameSizeCalculation=off
      link override defval: Value=KINP_ODOMETER_km_defval
      link override ovrdflg: Value=KINP_ODOMETER_km_ovrdflg
      link override ovrdval: Value=KINP_ODOMETER_km_ovrdval
  Terminator_1 : Terminator
  Terminator_2 : Terminator
  True_VHAL_METERKPHCalcu_kph : Constant  Value=TRUE  OutDataTypeStr=boolean
  True_VHAL_ODOMETER_km : Constant  Value=TRUE  OutDataTypeStr=boolean
  slr1_1 : BusSelector  OutputSignals=VINP_CANMsgValidMETER1_flg
  slr1_2 : BusSelector  OutputSignals=VINP_CANMsgValidMETER1_flg
  slr_VHAL_METERKPHCalcu_kph : BusSelector  OutputSignals=VHAL_METERKPHCalcu_kph
  slr_VHAL_ODOMETER_km : BusSelector  OutputSignals=VHAL_ODOMETER_km
  VINP_METERKPHCalcu_kph : Outport
  VINP_ODOMETER_km : Outport  Port=2
  wires:
  BHAL_outputs/1 -> [BHAL_outputs]
  inp_CanValid_bus/1 -> [inp_CanValid_bus]
  [BHAL_outputs] -> slr_VHAL_METERKPHCalcu_kph/1
  slr_VHAL_METERKPHCalcu_kph/1 -> METERKPHCalcu/1  "<VHAL_METERKPHCalcu_kph>"
  True_VHAL_METERKPHCalcu_kph/1 -> METERKPHCalcu/2
  [inp_CanValid_bus] -> slr1_1/1
  slr1_1/1 -> METERKPHCalcu/3  "<VINP_CANMsgValidMETER1_flg>"
  METERKPHCalcu/1 -> VINP_METERKPHCalcu_kph/1  "VINP_METERKPHCalcu_kph"
  METERKPHCalcu/2 -> Terminator_1/1
  [BHAL_outputs] -> slr_VHAL_ODOMETER_km/1
  slr_VHAL_ODOMETER_km/1 -> ODOMETER/1  "<VHAL_ODOMETER_km>"
  True_VHAL_ODOMETER_km/1 -> ODOMETER/2
  [inp_CanValid_bus] -> slr1_2/1
  slr1_2/1 -> ODOMETER/3  "<VINP_CANMsgValidMETER1_flg>"
  ODOMETER/1 -> VINP_ODOMETER_km/1  "VINP_ODOMETER_km"
  ODOMETER/2 -> Terminator_2/1

== system inp/INP/CAN3/SignalCheck/BMS1 ==
  BHAL_outputs : Inport
  inp_CanValid_bus : Inport  Port=2
  BMSChckSum1 : FVT_lib/inp/can_signal_template  SystemSampleTime=-1  VariantActivationTime=update diagram  Latency=0  AutoFrameSizeCalculation=off
      link override defval: Value=KINP_BMSChckSum1_enum_defval
      link override ovrdflg: Value=KINP_BMSChckSum1_enum_ovrdflg
      link override ovrdval: Value=KINP_BMSChckSum1_enum_ovrdval
  BMSRolCnct1 : FVT_lib/inp/can_signal_template  SystemSampleTime=-1  VariantActivationTime=update diagram  Latency=0  AutoFrameSizeCalculation=off
      link override defval: Value=KINP_BMSRolCnct1_enum_defval
      link override ovrdflg: Value=KINP_BMSRolCnct1_enum_ovrdflg
      link override ovrdval: Value=KINP_BMSRolCnct1_enum_ovrdval
  HVBPwrAvailChrg : FVT_lib/inp/can_signal_template  SystemSampleTime=-1  VariantActivationTime=update diagram  Latency=0  AutoFrameSizeCalculation=off
      link override defval: Value=KINP_HVBPwrAvailChrg_kW_defval
      link override ovrdflg: Value=KINP_HVBPwrAvailChrg_kW_ovrdflg
      link override ovrdval: Value=KINP_HVBPwrAvailChrg_kW_ovrdval
  HVBPwrAvailChrg30 : FVT_lib/inp/can_signal_template  SystemSampleTime=-1  VariantActivationTime=update diagram  Latency=0  AutoFrameSizeCalculation=off
      link override defval: Value=KINP_HVBPwrAvailChrg30_kW_defval
      link override ovrdflg: Value=KINP_HVBPwrAvailChrg30_kW_ovrdflg
      link override ovrdval: Value=KINP_HVBPwrAvailChrg30_kW_ovrdval
  HVBPwrAvailChrg60 : FVT_lib/inp/can_signal_template  SystemSampleTime=-1  VariantActivationTime=update diagram  Latency=0  AutoFrameSizeCalculation=off
      link override defval: Value=KINP_HVBPwrAvailChrg60_kW_defval
      link override ovrdflg: Value=KINP_HVBPwrAvailChrg60_kW_ovrdflg
      link override ovrdval: Value=KINP_HVBPwrAvailChrg60_kW_ovrdval
  HVBPwrAvailDchrg : FVT_lib/inp/can_signal_template  SystemSampleTime=-1  VariantActivationTime=update diagram  Latency=0  AutoFrameSizeCalculation=off
      link override defval: Value=KINP_HVBPwrAvailDchrg_kW_defval
      link override ovrdflg: Value=KINP_HVBPwrAvailDchrg_kW_ovrdflg
      link override ovrdval: Value=KINP_HVBPwrAvailDchrg_kW_ovrdval
  HVBPwrAvailDchrg30 : FVT_lib/inp/can_signal_template  SystemSampleTime=-1  VariantActivationTime=update diagram  Latency=0  AutoFrameSizeCalculation=off
      link override defval: Value=KINP_HVBPwrAvailDchrg30_kW_defval
      link override ovrdflg: Value=KINP_HVBPwrAvailDchrg30_kW_ovrdflg
      link override ovrdval: Value=KINP_HVBPwrAvailDchrg30_kW_ovrdval
  HVBPwrAvailDchrg60 : FVT_lib/inp/can_signal_template  SystemSampleTime=-1  VariantActivationTime=update diagram  Latency=0  AutoFrameSizeCalculation=off
      link override defval: Value=KINP_HVBPwrAvailDchrg60_kW_defval
      link override ovrdflg: Value=KINP_HVBPwrAvailDchrg60_kW_ovrdflg
      link override ovrdval: Value=KINP_HVBPwrAvailDchrg60_kW_ovrdval
  HVBattCurr : FVT_lib/inp/can_signal_template  SystemSampleTime=-1  VariantActivationTime=update diagram  Latency=0  AutoFrameSizeCalculation=off
      link override defval: Value=KINP_HVBattCurr_A_defval
      link override ovrdflg: Value=KINP_HVBattCurr_A_ovrdflg
      link override ovrdval: Value=KINP_HVBattCurr_A_ovrdval
  HVBattVolt : FVT_lib/inp/can_signal_template  SystemSampleTime=-1  VariantActivationTime=update diagram  Latency=0  AutoFrameSizeCalculation=off
      link override defval: Value=KINP_HVBattVolt_V_defval
      link override ovrdflg: Value=KINP_HVBattVolt_V_ovrdflg
      link override ovrdval: Value=KINP_HVBattVolt_V_ovrdval
  Terminator_{1..10} (10 alike) : Terminator
  True_VHAL_BMSChckSum1_enum : Constant  Value=TRUE  OutDataTypeStr=boolean
  True_VHAL_BMSRolCnct1_enum : Constant  Value=TRUE  OutDataTypeStr=boolean
  True_VHAL_HVBPwrAvailChrg30_kW : Constant  Value=TRUE  OutDataTypeStr=boolean
  True_VHAL_HVBPwrAvailChrg60_kW : Constant  Value=TRUE  OutDataTypeStr=boolean
  True_VHAL_HVBPwrAvailChrg_kW : Constant  Value=TRUE  OutDataTypeStr=boolean
  True_VHAL_HVBPwrAvailDchrg30_kW : Constant  Value=TRUE  OutDataTypeStr=boolean
  True_VHAL_HVBPwrAvailDchrg60_kW : Constant  Value=TRUE  OutDataTypeStr=boolean
  True_VHAL_HVBPwrAvailDchrg_kW : Constant  Value=TRUE  OutDataTypeStr=boolean
  True_VHAL_HVBattCurr_A : Constant  Value=TRUE  OutDataTypeStr=boolean
  True_VHAL_HVBattVolt_V : Constant  Value=TRUE  OutDataTypeStr=boolean
  slr1_{1..10} (10 alike) : BusSelector  OutputSignals=VINP_CANMsgValidBMS1_flg
  slr_VHAL_BMSChckSum1_enum : BusSelector  OutputSignals=VHAL_BMSChckSum1_enum
  slr_VHAL_BMSRolCnct1_enum : BusSelector  OutputSignals=VHAL_BMSRolCnct1_enum
  slr_VHAL_HVBPwrAvailChrg30_kW : BusSelector  OutputSignals=VHAL_HVBPwrAvailChrg30_kW
  slr_VHAL_HVBPwrAvailChrg60_kW : BusSelector  OutputSignals=VHAL_HVBPwrAvailChrg60_kW
  slr_VHAL_HVBPwrAvailChrg_kW : BusSelector  OutputSignals=VHAL_HVBPwrAvailChrg_kW
  slr_VHAL_HVBPwrAvailDchrg30_kW : BusSelector  OutputSignals=VHAL_HVBPwrAvailDchrg30_kW
  slr_VHAL_HVBPwrAvailDchrg60_kW : BusSelector  OutputSignals=VHAL_HVBPwrAvailDchrg60_kW
  slr_VHAL_HVBPwrAvailDchrg_kW : BusSelector  OutputSignals=VHAL_HVBPwrAvailDchrg_kW
  slr_VHAL_HVBattCurr_A : BusSelector  OutputSignals=VHAL_HVBattCurr_A
  slr_VHAL_HVBattVolt_V : BusSelector  OutputSignals=VHAL_HVBattVolt_V
  VINP_BMSChckSum1_enum : Outport
  VINP_BMSRolCnct1_enum : Outport  Port=2
  VINP_HVBPwrAvailChrg_kW : Outport  Port=3
  VINP_HVBPwrAvailChrg30_kW : Outport  Port=4
  VINP_HVBPwrAvailChrg60_kW : Outport  Port=5
  VINP_HVBPwrAvailDchrg_kW : Outport  Port=6
  VINP_HVBPwrAvailDchrg30_kW : Outport  Port=7
  VINP_HVBPwrAvailDchrg60_kW : Outport  Port=8
  VINP_HVBattCurr_A : Outport  Port=9
  VINP_HVBattVolt_V : Outport  Port=10
  wires:
  BHAL_outputs/1 -> [BHAL_outputs]
  inp_CanValid_bus/1 -> [inp_CanValid_bus]
  [BHAL_outputs] -> slr_VHAL_BMSChckSum1_enum/1
  slr_VHAL_BMSChckSum1_enum/1 -> BMSChckSum1/1  "<VHAL_BMSChckSum1_enum>"
  True_VHAL_BMSChckSum1_enum/1 -> BMSChckSum1/2
  [inp_CanValid_bus] -> slr1_1/1
  slr1_1/1 -> BMSChckSum1/3  "<VINP_CANMsgValidBMS1_flg>"
  BMSChckSum1/1 -> VINP_BMSChckSum1_enum/1  "VINP_BMSChckSum1_enum"
  BMSChckSum1/2 -> Terminator_1/1
  [BHAL_outputs] -> slr_VHAL_BMSRolCnct1_enum/1
  slr_VHAL_BMSRolCnct1_enum/1 -> BMSRolCnct1/1  "<VHAL_BMSRolCnct1_enum>"
  True_VHAL_BMSRolCnct1_enum/1 -> BMSRolCnct1/2
  [inp_CanValid_bus] -> slr1_2/1
  slr1_2/1 -> BMSRolCnct1/3  "<VINP_CANMsgValidBMS1_flg>"
  BMSRolCnct1/1 -> VINP_BMSRolCnct1_enum/1  "VINP_BMSRolCnct1_enum"
  BMSRolCnct1/2 -> Terminator_2/1
  [BHAL_outputs] -> slr_VHAL_HVBPwrAvailChrg_kW/1
  slr_VHAL_HVBPwrAvailChrg_kW/1 -> HVBPwrAvailChrg/1  "<VHAL_HVBPwrAvailChrg_kW>"
  True_VHAL_HVBPwrAvailChrg_kW/1 -> HVBPwrAvailChrg/2
  [inp_CanValid_bus] -> slr1_3/1
  slr1_3/1 -> HVBPwrAvailChrg/3  "<VINP_CANMsgValidBMS1_flg>"
  HVBPwrAvailChrg/1 -> VINP_HVBPwrAvailChrg_kW/1  "VINP_HVBPwrAvailChrg_kW"
  HVBPwrAvailChrg/2 -> Terminator_3/1
  [BHAL_outputs] -> slr_VHAL_HVBPwrAvailChrg30_kW/1
  slr_VHAL_HVBPwrAvailChrg30_kW/1 -> HVBPwrAvailChrg30/1  "<VHAL_HVBPwrAvailChrg30_kW>"
  True_VHAL_HVBPwrAvailChrg30_kW/1 -> HVBPwrAvailChrg30/2
  [inp_CanValid_bus] -> slr1_4/1
  slr1_4/1 -> HVBPwrAvailChrg30/3  "<VINP_CANMsgValidBMS1_flg>"
  HVBPwrAvailChrg30/1 -> VINP_HVBPwrAvailChrg30_kW/1  "VINP_HVBPwrAvailChrg30_kW"
  HVBPwrAvailChrg30/2 -> Terminator_4/1
  [BHAL_outputs] -> slr_VHAL_HVBPwrAvailChrg60_kW/1
  slr_VHAL_HVBPwrAvailChrg60_kW/1 -> HVBPwrAvailChrg60/1  "<VHAL_HVBPwrAvailChrg60_kW>"
  True_VHAL_HVBPwrAvailChrg60_kW/1 -> HVBPwrAvailChrg60/2
  [inp_CanValid_bus] -> slr1_5/1
  slr1_5/1 -> HVBPwrAvailChrg60/3  "<VINP_CANMsgValidBMS1_flg>"
  HVBPwrAvailChrg60/1 -> VINP_HVBPwrAvailChrg60_kW/1  "VINP_HVBPwrAvailChrg60_kW"
  HVBPwrAvailChrg60/2 -> Terminator_5/1
  [BHAL_outputs] -> slr_VHAL_HVBPwrAvailDchrg_kW/1
  slr_VHAL_HVBPwrAvailDchrg_kW/1 -> HVBPwrAvailDchrg/1  "<VHAL_HVBPwrAvailDchrg_kW>"
  True_VHAL_HVBPwrAvailDchrg_kW/1 -> HVBPwrAvailDchrg/2
  [inp_CanValid_bus] -> slr1_6/1
  slr1_6/1 -> HVBPwrAvailDchrg/3  "<VINP_CANMsgValidBMS1_flg>"
  HVBPwrAvailDchrg/1 -> VINP_HVBPwrAvailDchrg_kW/1  "VINP_HVBPwrAvailDchrg_kW"
  HVBPwrAvailDchrg/2 -> Terminator_6/1
  [BHAL_outputs] -> slr_VHAL_HVBPwrAvailDchrg30_kW/1
  slr_VHAL_HVBPwrAvailDchrg30_kW/1 -> HVBPwrAvailDchrg30/1  "<VHAL_HVBPwrAvailDchrg30_kW>"
  True_VHAL_HVBPwrAvailDchrg30_kW/1 -> HVBPwrAvailDchrg30/2
  [inp_CanValid_bus] -> slr1_7/1
  slr1_7/1 -> HVBPwrAvailDchrg30/3  "<VINP_CANMsgValidBMS1_flg>"
  HVBPwrAvailDchrg30/1 -> VINP_HVBPwrAvailDchrg30_kW/1  "VINP_HVBPwrAvailDchrg30_kW"
  HVBPwrAvailDchrg30/2 -> Terminator_7/1
  [BHAL_outputs] -> slr_VHAL_HVBPwrAvailDchrg60_kW/1
  slr_VHAL_HVBPwrAvailDchrg60_kW/1 -> HVBPwrAvailDchrg60/1  "<VHAL_HVBPwrAvailDchrg60_kW>"
  True_VHAL_HVBPwrAvailDchrg60_kW/1 -> HVBPwrAvailDchrg60/2
  [inp_CanValid_bus] -> slr1_8/1
  slr1_8/1 -> HVBPwrAvailDchrg60/3  "<VINP_CANMsgValidBMS1_flg>"
  HVBPwrAvailDchrg60/1 -> VINP_HVBPwrAvailDchrg60_kW/1  "VINP_HVBPwrAvailDchrg60_kW"
  HVBPwrAvailDchrg60/2 -> Terminator_8/1
  [BHAL_outputs] -> slr_VHAL_HVBattCurr_A/1
  slr_VHAL_HVBattCurr_A/1 -> HVBattCurr/1  "<VHAL_HVBattCurr_A>"
  True_VHAL_HVBattCurr_A/1 -> HVBattCurr/2
  [inp_CanValid_bus] -> slr1_9/1
  slr1_9/1 -> HVBattCurr/3  "<VINP_CANMsgValidBMS1_flg>"
  HVBattCurr/1 -> VINP_HVBattCurr_A/1  "VINP_HVBattCurr_A"
  HVBattCurr/2 -> Terminator_9/1
  [BHAL_outputs] -> slr_VHAL_HVBattVolt_V/1
  slr_VHAL_HVBattVolt_V/1 -> HVBattVolt/1  "<VHAL_HVBattVolt_V>"
  True_VHAL_HVBattVolt_V/1 -> HVBattVolt/2
  [inp_CanValid_bus] -> slr1_10/1
  slr1_10/1 -> HVBattVolt/3  "<VINP_CANMsgValidBMS1_flg>"
  HVBattVolt/1 -> VINP_HVBattVolt_V/1  "VINP_HVBattVolt_V"
  HVBattVolt/2 -> Terminator_10/1
